simulink model "kolbenfcn"  (R2018b)
settings: Solver=VariableStepAuto  StartTime=0.0  StopTime=10  RelTol=10e-3
values from neighbouring files (symbols this model uses):
  AK = pi/4 * dK^2    (= 0.000314159265359)    [lab3_teil2.m]    (also in lab3_teil3.m; modelbildung_lab3.m)
  FR = 5    [lab3_teil2.m]    (also in lab3_teil3.m; modelbildung_lab3.m)
  m = 1    [lab3_teil2.m]    (also in lab3_teil3.m; modelbildung_lab3.m)
  rho = 850    [lab3_teil2.m]    (also in lab3_teil3.m; modelbildung_lab3.m)
  zeta = 0.5    [lab3_teil2.m]    (also in lab3_teil3.m; modelbildung_lab3.m)
libraries: simulink x2
settings Model: Creator=st172720  LastModifiedBy=Naveen
settings DebuggingCC: LibraryContextMissingDiagnostic=none
settings SFSimCC: SimUseLocalCustomCode=off
settings RTWCC: RTWUseLocalCustomCode=off

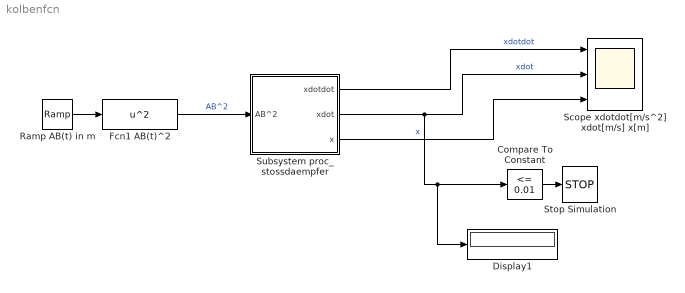
== system kolbenfcn ==
  Compare To Constant : simulink/Logic and Bit Operations/Compare To Constant  relop=<=  const=0.01  OutDataTypeStr=boolean
  Display1 : Display
  Fcn1 AB(t)^2 : Fcn  Expr=u^2
  Ramp AB(t) in m : simulink/Sources/Ramp  slope=-4.5e-5/0.05  start=0.05  InitialOutput=- 4.5e-5
  Scope xdotdot[m/s^2] xdot[m/s] x[m] : Scope  NumInputPorts=3
  Stop Simulation : Stop
  Subsystem proc_stossdaempfer : Subsystem
  wires:
  Fcn1 AB(t)^2/1 -> Subsystem proc_stossdaempfer/1(AB^2)  "AB^2"
  Subsystem proc_stossdaempfer/1(xdotdot) -> Scope xdotdot[m/s^2] xdot[m/s] x[m]/1  "xdotdot"
  Subsystem proc_stossdaempfer/2(xdot) -> Compare To Constant/1, Display1/1, Scope xdotdot[m/s^2] xdot[m/s] x[m]/2  "xdot"
  Subsystem proc_stossdaempfer/3(x) -> Scope xdotdot[m/s^2] xdot[m/s] x[m]/3  "x"
  Compare To Constant/1 -> Stop Simulation/1
  Ramp AB(t) in m/1 -> Fcn1 AB(t)^2/1

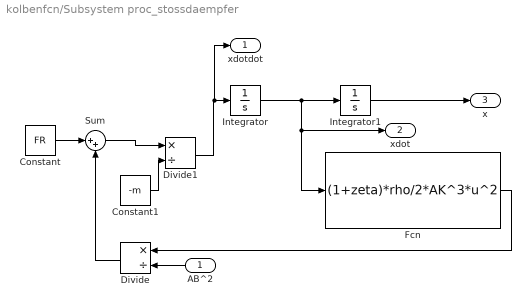
== system kolbenfcn/Subsystem proc_stossdaempfer ==
  AB^2 : Inport
  Constant : Constant  Value=FR
  Constant1 : Constant  Value=-m
  Divide : Product  Inputs=*/
  Divide1 : Product  Inputs=*/
  Fcn : Fcn  Expr=(1+zeta)*rho/2*AK^3*u^2
  Integrator : Integrator  InitialCondition=3
  Integrator1 : Integrator
  Sum : Sum  Inputs=|++
  xdotdot : Outport
  xdot : Outport  Port=2
  x : Outport  Port=3
  wires:
  Integrator/1 -> Fcn/1, xdot/1, Integrator1/1
  Divide/1 -> Sum/2
  Constant1/1 -> Divide1/2
  Constant/1 -> Sum/1
  Divide1/1 -> xdotdot/1, Integrator/1
  Fcn/1 -> Divide/1
  Sum/1 -> Divide1/1
  Integrator1/1 -> x/1
  AB^2/1 -> Divide/2
